simulink model "Sim_Knickarmroboter_AndreasPaul"  (R2024a)
settings: Solver=VariableStepAuto  StartTime=0.0  StopTime=10.0  RelTol=1e-3
libraries: slpidlib x1
settings Model: Creator=apaul  LastModifiedBy=apaul

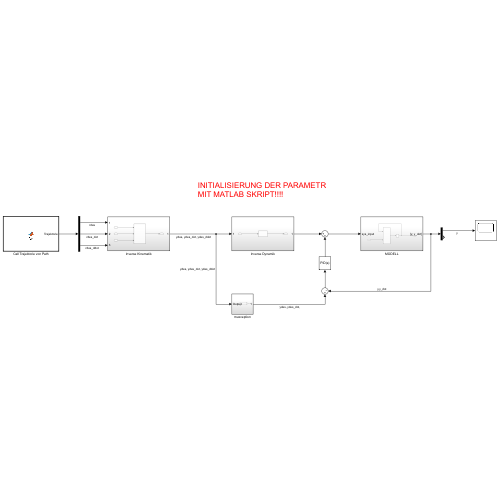
[thumbnail: Simulink's stored preview of the top-level diagram]
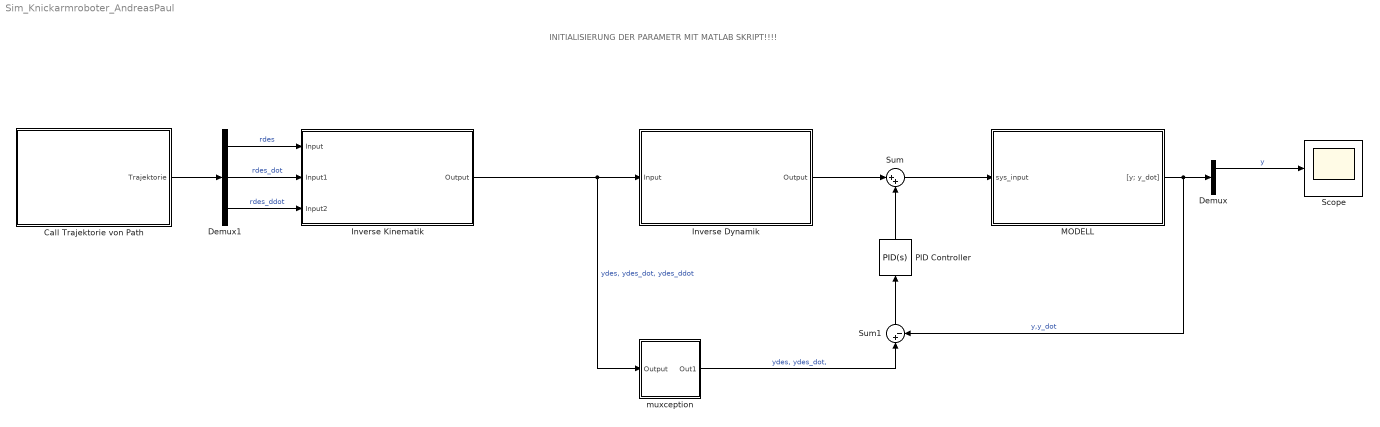
== system Sim_Knickarmroboter_AndreasPaul ==
  note: INITIALISIERUNG DER PARAMETR MIT MATLAB SKRIPT!!!!
  Call Trajektorie von Path : MATLAB Function  TreatAsAtomicUnit=on
  Demux : Demux  Outputs=2
  Demux1 : Demux  Outputs=3
  Inverse Dynamik : Subsystem
  Inverse Kinematik : Subsystem
  MODELL : Subsystem
  PID Controller : slpidlib/PID Controller  Controller=PID  Form=Parallel  TimeDomain=Continuous-time  UseExternalTs=off  SampleTime=-1  IntegratorMethod=Forward Euler  FilterMethod=Forward Euler  ControllerParametersSource=internal  P=1  I=1  UseKiTs=off  D=0  UseExternalDerivativeSource=off  N=100  UseFilter=on  TunerSelectOption=Transfer Function Based (PID Tuner App)  InitialConditionSource=internal  InitialConditionForIntegrator=0  InitialConditionForFilter=0  DifferentiatorICPrevScaledInput=0  ExternalReset=none  TrackingMode=off  Kt=1  LimitOutput=off  SatLimitsSource=internal  UpperSaturationLimit=inf  LowerSaturationLimit=-inf  LinearizeAsGain=on  AntiWindupMode=none  Kb=1  LimitIntegrator=off  UpperIntegratorSaturationLimit=inf  LowerIntegratorSaturationLimit=-inf  POutMin=[]  POutMax=[]  IOutMin=[]  IOutMax=[]  DOutMin=[]  DOutMax=[]  NOutMin=[]  NOutMax=[]  SumOutMin=[]  SumOutMax=[]  SaturationOutMin=[]  SaturationOutMax=[]  PParamMin=[]  PParamMax=[]  IParamMin=[]  IParamMax=[]  DParamMin=[]  DParamMax=[]  NParamMin=[]  NParamMax=[]  KbParamMin=[]  KbParamMax=[]  KtParamMin=[]  KtParamMax=[]  KbOutMin=[]  KbOutMax=[]  KtOutMin=[]  KtOutMax=[]  IntegratorOutMin=[]  IntegratorOutMax=[]  FilterOutMin=[]  FilterOutMax=[]  SumI1OutMin=[]  SumI1OutMax=[]  SumI2OutMin=[]  SumI2OutMax=[]  SumI3OutMin=[]  SumI3OutMax=[]  SumI4OutMin=[]  SumI4OutMax=[]  SumDOutMin=[]  SumDOutMax=[]  DifferentiatorOutMin=[]  DifferentiatorOutMax=[]  FilterDiffOutCoefMin=[]  FilterDiffOutCoefMax=[]  ReciprocalOutMin=[]  ReciprocalOutMax=[]  SumDenOutMin=[]  SumDenOutMax=[]  SumNumOutMin=[]  SumNumOutMax=[]  DivideOutMin=[]  DivideOutMax=[]  UdiffTsProdOutMin=[]  UdiffTsProdOutMax=[]  NTsProdOutMin=[]  NTsProdOutMax=[]  UintegralTsProdOutMin=[]  UintegralTsProdOutMax=[]  UngainTsProdOutMin=[]  UngainTsProdOutMax=[]  ClampingZeroOutDataTypeStr=Inherit: Inherit via back propagation  ClampingZeroOutMin=[]  ClampingZeroOutMax=[]  FilterDenConstantOutDataTypeStr=Inherit: Inherit via back propagation  FilterDenConstantOutMin=[]  FilterDenConstantOutMax=[]  PCopyOutDataTypeStr=Inherit: Inherit via back propagation  PCopyOutMin=[]  PCopyOutMax=[]  NCopyOutDataTypeStr=Inherit: Inherit via back propagation  NCopyOutMin=[]  NCopyOutMax=[]  IntegratorContinuousStateAttributes=''  IntegratorStateMustResolveToSignalObject=off  IntegratorRTWStateStorageClass=Auto  FilterContinuousStateAttributes=''  FilterStateMustResolveToSignalObject=off  FilterRTWStateStorageClass=Auto  ParallelPVariant=InternalParameters  IdealPVariant=Disabled  IVariant=InternalParameters  DVariant=InternalParameters  IntegratorVariant=Continuous  SatVariant=Disabled  AWVariant=Passthrough  PCopyVariant=Disabled  TRVariant=Disabled  FdbkBlocksVariant=Forward  IdealPFdbkVariant=Disabled  SatFdbkVariant=Disabled  DerivativeFilterVariant=ContFilter  NVariant=InternalParameters  NCopyVariant=Disabled  FilterICVariant=InternalICsFilter  IntegratorICVariant=InternalICs  ExternalResetVariant=Disabled  TRSumVariant=Passthrough  SumFdbkVariant=Disabled  SumVariant=Sum_PID  TsampFilterVariant=InternalTs  TsampNgainVariant=Passthrough  TsampIntegralVariant=Passthrough  ExternalSaturationOutDataTypeStr=Inherit: Same as second input  DerivativeSourceVariant=ErrorSignal
  Scope : Scope
  Sum : Sum  Inputs=|++
  Sum1 : Sum  Inputs=|+-
  muxception : Subsystem
  wires:
  Sum/1 -> MODELL/1(sys_input)
  PID Controller/1 -> Sum/2
  Sum1/1 -> PID Controller/1
  MODELL/1("[y; y_dot]") -> Demux/1, Sum1/2  "y,y_dot"
  Inverse Kinematik/1(Output) -> Inverse Dynamik/1(Input), muxception/1(Output)  "ydes, ydes_dot, ydes_ddot"
  Inverse Dynamik/1(Output) -> Sum/1
  Demux/1 -> Scope/1  "y"
  muxception/1(Out1) -> Sum1/1  "ydes, ydes_dot,"
  Call Trajektorie von Path/1(Trajektorie) -> Demux1/1
  Demux1/3 -> Inverse Kinematik/3(Input2)  "rdes_ddot"
  Demux1/2 -> Inverse Kinematik/2(Input1)  "rdes_dot"
  Demux1/1 -> Inverse Kinematik/1(Input)  "rdes"

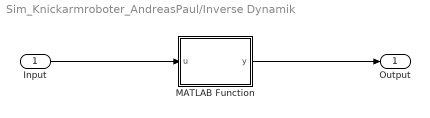
== system Sim_Knickarmroboter_AndreasPaul/Inverse Dynamik ==
  Input : Inport
  MATLAB Function : MATLAB Function  TreatAsAtomicUnit=on
  Output : Outport
  wires:
  Input/1 -> MATLAB Function/1(u)
  MATLAB Function/1(y) -> Output/1

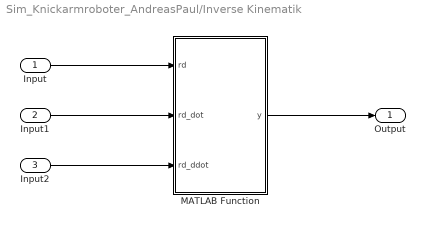
== system Sim_Knickarmroboter_AndreasPaul/Inverse Kinematik ==
  Input : Inport
  Input1 : Inport  Port=2
  Input2 : Inport  Port=3
  MATLAB Function : MATLAB Function  TreatAsAtomicUnit=on
  Output : Outport
  wires:
  Input/1 -> MATLAB Function/1(rd)
  MATLAB Function/1(y) -> Output/1
  Input1/1 -> MATLAB Function/2(rd_dot)
  Input2/1 -> MATLAB Function/3(rd_ddot)

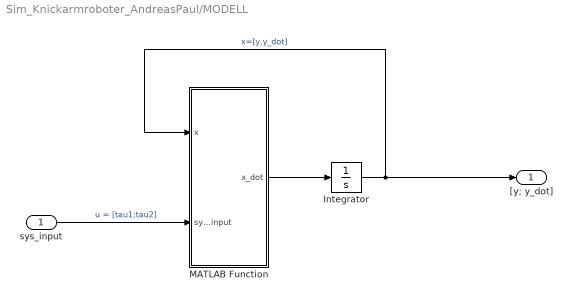
== system Sim_Knickarmroboter_AndreasPaul/MODELL ==
  sys_input : Inport
  Integrator : Integrator
  MATLAB Function : MATLAB Function  TreatAsAtomicUnit=on
  "[y; y_dot]" : Outport
  wires:
  MATLAB Function/1(x_dot) -> Integrator/1
  Integrator/1 -> "[y; y_dot]"/1, MATLAB Function/1(x)  "x=[y,y_dot]"
  sys_input/1 -> MATLAB Function/2(sys_input)  "u = [tau1;tau2]"

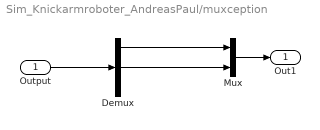
== system Sim_Knickarmroboter_AndreasPaul/muxception ==
  Output : Inport
  Demux : Demux  Outputs=3
  Mux : Mux  Inputs=2
  Out1 : Outport
  wires:
  Output/1 -> Demux/1
  Demux/1 -> Mux/1
  Demux/2 -> Mux/2
  Mux/1 -> Out1/1

== matlab function Sim_Knickarmroboter_AndreasPaul/Inverse Dynamik/MATLAB Function ==
  data: u input; y output
function y = fcn(u)

y = u;

== matlab function Sim_Knickarmroboter_AndreasPaul/MODELL/MATLAB Function ==
  data: x input; x_dot output; sys_input input
function x_dot = fcn(x, sys_input)

end

== matlab function Sim_Knickarmroboter_AndreasPaul/Inverse Kinematik/MATLAB Function ==
  data: rd input; y output; rd_dot input; rd_ddot input
function y = fcn(rd,rd_dot,rd_ddot)

y = u;

== matlab function Sim_Knickarmroboter_AndreasPaul/Call Trajektorie von Path ==
  data: Trajektorie output
function Trajektorie = fcn()

%CALL HERE TRAJECTORIES FROM PATH

Trajektorie = u;
